simulink model "mars_rover_ex_1b_22b"  (R2022b)
settings: Solver=ode23t  StartTime=0.0  StopTime=Rover.simStopTimeEx1b  FixedStep=1e-2  MaxStep=0.05  RelTol=1e-3  AbsTol=1e-3  EnableMultiTasking=on
StartFcn:
  | mars_rover_ex1b_sim_callback
model workspace (MATLAB code in the model file):
  | addpath("mars_rover_helpers");
  | % Load Rover Arm model for IK
  | mdlpath = ['mars_rover_data',filesep,'mars_rover_arm'];
  | load_system(mdlpath);
  | 
  | imdata = zeros(3,3,3);
  | 
  | % Temp
  | Kp_steer = 1;
  | Ki_steer = 1;
  | Kd_steer = 1;
  | 
  | Kp = 1;
  | Ki = 1;
  | Kd = 1;
values from neighbouring files (symbols this model uses):
  cam_base_angle = 0    [mars_rover_params.m]
  cam_target_angle = 20    [mars_rover_params.m]
  mapData = false(197,200)    [mars_rover_params.m]    (also in mars_rover_startup.m)
  roverPath = app.rover_path    [NavigateOnMars.m]    (also in mars_rover_params.m = rover_path1)
undefined symbols (not defined in the file or in its folder): Arm, armJointAng, armJointTrqs, cameraData, eeConfig, pose, Rover, sampleLocation, steerAng, steerTrqs, Terrain, vSpeed, Wheel1_G, Wheel2_G, Wheel3_G, Wheel4_G, Wheel5_G, Wheel6_G, wheelTrqs, wSpeeds, X, Y, Z
libraries: sm_lib x238, nesl_utility x80, slpidlib x3, simulink x3, simulink_extras x2, robotcorelib x1, robotalgslib x1
(part 5 of 9)

== system mars_rover_ex_1b_22b/Perception/navCamSubsystem/rsm_lower_mast_2_RIGID ==
  note: 15 deg offset
  Cylindrical Solid : sm_lib/Body Elements/Cylindrical Solid  GraphicAmbientColor=[0.15 0.15 0.15 1.0]  BasedOnType=Density  CenterOfMass=[0 0 0]  CenterOfMassUnits=m  GraphicDiffuseColor=[1 1 0.8]  CylinderLength=3.5/10  CylinderLengthUnits=m  CylinderRadius=0.4/10  CylinderRadiusUnits=m  Density=1000  DensityUnits=kg/m^3  DoExposeReferenceFrame=on  GraphicEmissiveColor=[0.0 0.0 0.0 1.0]  ExportEntireGeometry=off  SerializedFrames=<Frames><Frame><Id>Frame1</Id><Value><Name>F1</Name><Origin><Source>GeometricFeature</Source><FeatureName>bottom surface</FeatureName></Origin><PrimaryAxis><DefinedDirection>+Z</DefinedDirection><Source>ReferenceFrame</Source><SourceDirection>+X</SourceDirection><FeatureName></FeatureName></PrimaryAxis><SecondaryAxis><DefinedDirection>+X</DefinedDirection><Source>ReferenceFrame</Source><SourceDirection>+Z</SourceDirection><FeatureName></FeatureName></SecondaryAxis></Value></Frame><Frame><Id>Frame2</Id><Value><Name>F2</Name><Origin><Source>GeometricFeature</Source><FeatureName>top surface</FeatureName></Origin><PrimaryAxis><DefinedDirection>+Z</DefinedDirection><Source>ReferenceFrame</Source><SourceDirection>+Z</SourceDirection><FeatureName></FeatureName></PrimaryAxis><SecondaryAxis><DefinedDirection>+X</DefinedDirection><Source>ReferenceFrame</Source><SourceDirection>+X</SourceDirection><FeatureName></FeatureName></SecondaryAxis></Value></Frame></Frames>  MarkerShape=Sphere  MarkerSize=10  GraphicType=FromGeometry  InertiaType=CalculateFromGeometry  Mass=1  MassUnits=kg  MomentsOfInertia=[1 1 1]  MomentsOfInertiaUnits=kg*m^2  GraphicOpacity=1.0  ProductsOfInertia=[0 0 0]  ProductsOfInertiaUnits=kg*m^2  GraphicShininess=75  GraphicSpecularColor=[0.5 0.5 0.5 1.0]  GraphicVisPropType=SimpleVisualProperties
  Cylindrical Solid1 : sm_lib/Body Elements/Cylindrical Solid  GraphicAmbientColor=[0.15 0.15 0.15 1.0]  BasedOnType=Density  CenterOfMass=[0 0 0]  CenterOfMassUnits=m  GraphicDiffuseColor=[1 1 0.8]  CylinderLength=0.85/10  CylinderLengthUnits=m  CylinderRadius=0.6/10  CylinderRadiusUnits=m  Density=1000  DensityUnits=kg/m^3  DoExposeReferenceFrame=on  GraphicEmissiveColor=[0.0 0.0 0.0 1.0]  ExportEntireGeometry=off  SerializedFrames=<Frames><Frame><Id>Frame1</Id><Value><Name>F1</Name><Origin><Source>GeometricFeature</Source><FeatureName>bottom surface</FeatureName></Origin><PrimaryAxis><DefinedDirection>+Z</DefinedDirection><Source>ReferenceFrame</Source><SourceDirection>+Z</SourceDirection><FeatureName></FeatureName></PrimaryAxis><SecondaryAxis><DefinedDirection>+X</DefinedDirection><Source>ReferenceFrame</Source><SourceDirection>+X</SourceDirection><FeatureName></FeatureName></SecondaryAxis></Value></Frame></Frames>  MarkerShape=Sphere  MarkerSize=10  GraphicType=FromGeometry  InertiaType=CalculateFromGeometry  Mass=1  MassUnits=kg  MomentsOfInertia=[1 1 1]  MomentsOfInertiaUnits=kg*m^2  GraphicOpacity=1.0  ProductsOfInertia=[0 0 0]  ProductsOfInertiaUnits=kg*m^2  GraphicShininess=75  GraphicSpecularColor=[0.5 0.5 0.5 1.0]  GraphicVisPropType=SimpleVisualProperties
  Cylindrical Solid2 : sm_lib/Body Elements/Cylindrical Solid  GraphicAmbientColor=[0.15 0.15 0.15 1.0]  BasedOnType=Density  CenterOfMass=[0 0 0]  CenterOfMassUnits=m  GraphicDiffuseColor=[1 1 0.8]  CylinderLength=0.2/10  CylinderLengthUnits=m  CylinderRadius=0.7/10  CylinderRadiusUnits=m  Density=1000  DensityUnits=kg/m^3  DoExposeReferenceFrame=on  GraphicEmissiveColor=[0.0 0.0 0.0 1.0]  ExportEntireGeometry=off  SerializedFrames=<Frames><Frame><Id>Frame1</Id><Value><Name>F1</Name><Origin><Source>GeometricFeature</Source><FeatureName>top surface</FeatureName></Origin><PrimaryAxis><DefinedDirection>+Z</DefinedDirection><Source>ReferenceFrame</Source><SourceDirection>+Z</SourceDirection><FeatureName></FeatureName></PrimaryAxis><SecondaryAxis><DefinedDirection>+X</DefinedDirection><Source>ReferenceFrame</Source><SourceDirection>+X</SourceDirection><FeatureName></FeatureName></SecondaryAxis></Value></Frame></Frames>  MarkerShape=Sphere  MarkerSize=10  GraphicType=FromGeometry  InertiaType=CalculateFromGeometry  Mass=1  MassUnits=kg  MomentsOfInertia=[1 1 1]  MomentsOfInertiaUnits=kg*m^2  GraphicOpacity=1.0  ProductsOfInertia=[0 0 0]  ProductsOfInertiaUnits=kg*m^2  GraphicShininess=75  GraphicSpecularColor=[0.5 0.5 0.5 1.0]  GraphicVisPropType=SimpleVisualProperties
  Cylindrical Solid3 : sm_lib/Body Elements/Cylindrical Solid  GraphicAmbientColor=[0.15 0.15 0.15 1.0]  BasedOnType=Density  CenterOfMass=[0 0 0]  CenterOfMassUnits=m  GraphicDiffuseColor=[1 1 0.8]  CylinderLength=1.25/10  CylinderLengthUnits=m  CylinderRadius=0.15/10  CylinderRadiusUnits=m  Density=2000  DensityUnits=kg/m^3  DoExposeReferenceFrame=off  GraphicEmissiveColor=[0.0 0.0 0.0 1.0]  ExportEntireGeometry=off  SerializedFrames=<Frames><Frame><Id>Frame1</Id><Value><Name>F1</Name><Origin><Source>GeometricFeature</Source><FeatureName>bottom surface</FeatureName></Origin><PrimaryAxis><DefinedDirection>+Z</DefinedDirection><Source>ReferenceFrame</Source><SourceDirection>+Z</SourceDirection><FeatureName></FeatureName></PrimaryAxis><SecondaryAxis><DefinedDirection>+X</DefinedDirection><Source>ReferenceFrame</Source><SourceDirection>+X</SourceDirection><FeatureName></FeatureName></SecondaryAxis></Value></Frame></Frames>  MarkerShape=Sphere  MarkerSize=10  GraphicType=FromGeometry  InertiaType=CalculateFromGeometry  Mass=1  MassUnits=kg  MomentsOfInertia=[1 1 1]  MomentsOfInertiaUnits=kg*m^2  GraphicOpacity=1.0  ProductsOfInertia=[0 0 0]  ProductsOfInertiaUnits=kg*m^2  GraphicShininess=75  GraphicSpecularColor=[0.5 0.5 0.5 1.0]  GraphicVisPropType=SimpleVisualProperties
  Cylindrical Solid4 : sm_lib/Body Elements/Cylindrical Solid  GraphicAmbientColor=[0.15 0.15 0.15 1.0]  BasedOnType=Density  CenterOfMass=[0 0 0]  CenterOfMassUnits=m  GraphicDiffuseColor=[1 1 0.8]  CylinderLength=1.5/10  CylinderLengthUnits=m  CylinderRadius=0.15/10  CylinderRadiusUnits=m  Density=2000  DensityUnits=kg/m^3  DoExposeReferenceFrame=off  GraphicEmissiveColor=[0.0 0.0 0.0 1.0]  ExportEntireGeometry=off  SerializedFrames=<Frames><Frame><Id>Frame1</Id><Value><Name>F1</Name><Origin><Source>GeometricFeature</Source><FeatureName>bottom surface</FeatureName></Origin><PrimaryAxis><DefinedDirection>+Z</DefinedDirection><Source>ReferenceFrame</Source><SourceDirection>+Z</SourceDirection><FeatureName></FeatureName></PrimaryAxis><SecondaryAxis><DefinedDirection>+X</DefinedDirection><Source>ReferenceFrame</Source><SourceDirection>+X</SourceDirection><FeatureName></FeatureName></SecondaryAxis></Value></Frame></Frames>  MarkerShape=Sphere  MarkerSize=10  GraphicType=FromGeometry  InertiaType=CalculateFromGeometry  Mass=1  MassUnits=kg  MomentsOfInertia=[1 1 1]  MomentsOfInertiaUnits=kg*m^2  GraphicOpacity=1.0  ProductsOfInertia=[0 0 0]  ProductsOfInertiaUnits=kg*m^2  GraphicShininess=75  GraphicSpecularColor=[0.5 0.5 0.5 1.0]  GraphicVisPropType=SimpleVisualProperties
  Rigid Transform : sm_lib/Frames and Transforms/Rigid Transform  TranslationMethod=StandardAxis  TranslationStandardOffset=-0.55  TranslationLengthUnit=cm  TranslationStandardAxis=+X  TranslationCartesianOffset=[0 0 0]  TranslationROffset=0  TranslationROffsetUnits=m  TranslationZOffset=0  TranslationZOffsetUnits=m  TranslationThetaOffset=0  TranslationThetaOffsetUnits=deg  RotationMethod=None  RotationAngleUnits=deg  RotationStandardAxis=+X  RotationAngle=75  RotationArbitraryAxis=[0 0 1]  FollAlignAxisA=+X  BaseAlignAxisA=+Y  FollAlignAxisB=+Y  BaseAlignAxisB=+Z  RotationSequenceAxes=FollowerAxes  RotationSequence=XYX  RotationSequenceAngles=[0 0 0]  RotationSequenceAnglesUnits=deg  RotationMatrix=[1 0 0; 0 1 0; 0 0 1]  Quaternion=[1 0 0 0]
  Rigid Transform1 : sm_lib/Frames and Transforms/Rigid Transform  TranslationMethod=Cartesian  TranslationStandardOffset=-0.55  TranslationLengthUnit=cm  TranslationStandardAxis=+X  TranslationCartesianOffset=[0 -0.3 1]  TranslationROffset=0  TranslationROffsetUnits=m  TranslationZOffset=0  TranslationZOffsetUnits=m  TranslationThetaOffset=0  TranslationThetaOffsetUnits=deg  RotationMethod=StandardAxis  RotationAngleUnits=deg  RotationStandardAxis=+X  RotationAngle=45  RotationArbitraryAxis=[0 0 1]  FollAlignAxisA=+X  BaseAlignAxisA=+Y  FollAlignAxisB=+Y  BaseAlignAxisB=+Z  RotationSequenceAxes=FollowerAxes  RotationSequence=ZYZ  RotationSequenceAngles=[0 -90 0]  RotationSequenceAnglesUnits=deg  RotationMatrix=[1 0 0; 0 1 0; 0 0 1]  Quaternion=[1 0 0 0]
  Rigid Transform2 : sm_lib/Frames and Transforms/Rigid Transform  TranslationMethod=Cartesian  TranslationStandardOffset=-0.55  TranslationLengthUnit=cm  TranslationStandardAxis=+X  TranslationCartesianOffset=[0 0.3 1]  TranslationROffset=0  TranslationROffsetUnits=m  TranslationZOffset=0  TranslationZOffsetUnits=m  TranslationThetaOffset=0  TranslationThetaOffsetUnits=deg  RotationMethod=StandardAxis  RotationAngleUnits=deg  RotationStandardAxis=+X  RotationAngle=-45  RotationArbitraryAxis=[0 0 1]  FollAlignAxisA=+X  BaseAlignAxisA=+Y  FollAlignAxisB=+Y  BaseAlignAxisB=+Z  RotationSequenceAxes=FollowerAxes  RotationSequence=ZYZ  RotationSequenceAngles=[0 90 0]  RotationSequenceAnglesUnits=deg  RotationMatrix=[1 0 0; 0 1 0; 0 0 1]  Quaternion=[1 0 0 0]
  Bottom : PMIOPort  Side=Left
  Top : PMIOPort  Port=2  Side=Right
  connections:
  Cylindrical Solid2/RConn1 -- Cylindrical Solid/LConn2
  Bottom/RConn1 -- Cylindrical Solid1/LConn1
  Top/RConn1 -- Cylindrical Solid2/LConn1
  Cylindrical Solid4/LConn1 -- Rigid Transform1/RConn1
  Rigid Transform/RConn1 -- Cylindrical Solid1/RConn1
  Rigid Transform/LConn1 -- Cylindrical Solid/LConn1
  Cylindrical Solid/RConn1 -- Rigid Transform2/LConn1 -- Rigid Transform1/LConn1
  Cylindrical Solid3/LConn1 -- Rigid Transform2/RConn1

== system mars_rover_ex_1b_22b/Perception/navCamSubsystem/rsm_outer_ring_1_RIGID ==
  Cylindrical Solid1 : sm_lib/Body Elements/Cylindrical Solid  GraphicAmbientColor=[0.15 0.15 0.15 1.0]  BasedOnType=Density  CenterOfMass=[0 0 0]  CenterOfMassUnits=m  GraphicDiffuseColor=[0.2 0.2 0.2]  CylinderLength=0.5/10  CylinderLengthUnits=m  CylinderRadius=0.9/10  CylinderRadiusUnits=m  Density=2000  DensityUnits=kg/m^3  DoExposeReferenceFrame=off  GraphicEmissiveColor=[0.0 0.0 0.0 1.0]  ExportEntireGeometry=off  SerializedFrames=<Frames><Frame><Id>Frame1</Id><Value><Name>F1</Name><Origin><Source>GeometricFeature</Source><FeatureName>bottom surface</FeatureName></Origin><PrimaryAxis><DefinedDirection>+Z</DefinedDirection><Source>ReferenceFrame</Source><SourceDirection>+Z</SourceDirection><FeatureName></FeatureName></PrimaryAxis><SecondaryAxis><DefinedDirection>+X</DefinedDirection><Source>ReferenceFrame</Source><SourceDirection>+X</SourceDirection><FeatureName></FeatureName></SecondaryAxis></Value></Frame><Frame><Id>Frame2</Id><Value><Name>F2</Name><Origin><Source>GeometricFeature</Source><FeatureName>top surface</FeatureName></Origin><PrimaryAxis><DefinedDirection>+Z</DefinedDirection><Source>ReferenceFrame</Source><SourceDirection>+Z</SourceDirection><FeatureName></FeatureName></PrimaryAxis><SecondaryAxis><DefinedDirection>+X</DefinedDirection><Source>ReferenceFrame</Source><SourceDirection>+X</SourceDirection><FeatureName></FeatureName></SecondaryAxis></Value></Frame></Frames>  MarkerShape=Sphere  MarkerSize=10  GraphicType=FromGeometry  InertiaType=CalculateFromGeometry  Mass=1  MassUnits=kg  MomentsOfInertia=[1 1 1]  MomentsOfInertiaUnits=kg*m^2  GraphicOpacity=1.0  ProductsOfInertia=[0 0 0]  ProductsOfInertiaUnits=kg*m^2  GraphicShininess=75  GraphicSpecularColor=[0.5 0.5 0.5 1.0]  GraphicVisPropType=SimpleVisualProperties
  F1 : PMIOPort  Side=Left
  F : PMIOPort  Port=2  Side=Left
  connections:
  F1/RConn1 -- Cylindrical Solid1/RConn1
  F/RConn1 -- Cylindrical Solid1/LConn1

== system mars_rover_ex_1b_22b/Perception/navCamSubsystem/rsm_upper_mast_1_RIGID ==
  In1 : Inport
  CamUpDown : sm_lib/Joints/Revolute Joint  JointMode=Normal  SenseConstraintForce=off  SenseConstraintForceX=off  SenseConstraintForceY=off  SenseConstraintForceZ=off  SenseConstraintTorque=off  SenseConstraintTorqueX=off  SenseConstraintTorqueY=off  SenseConstraintTorqueZ=off  SenseTotalForce=off  SenseTotalForceX=off  SenseTotalForceY=off  SenseTotalForceZ=off  SenseTotalTorque=off  SenseTotalTorqueX=off  SenseTotalTorqueY=off  SenseTotalTorqueZ=off  CompositeWrenchDir=FollowerOnBase  CompositeWrenchFrame=BaseFrame  EquilibriumPosition=0  EquilibriumPositionUnits=deg  SpringStiffness=0  SpringStiffnessUnits=N*m/deg  DampingCoefficient=0  DampingCoefficientUnits=N*m/(deg/s)  TorqueActuationMode=ComputedTorque  MotionActuationMode=InputMotion  SensePosition=off  SenseVelocity=off  SenseAcceleration=off  SenseTorqueForce=off  SenseLowerLimitTorqueForce=off  SenseUpperLimitTorqueForce=off  LowerLimitSpecify=off  LowerLimitBound=-90  LowerLimitBoundUnits=deg  LowerLimitStiffness=1e4  LowerLimitStiffnessUnits=N*m/deg  LowerLimitDamping=10  LowerLimitDampingUnits=N*m/(deg/s)  LowerLimitTransitionRegionWidth=0.1  LowerLimitTransitionRegionWidthUnits=deg  UpperLimitSpecify=off  UpperLimitBound=90  UpperLimitBoundUnits=deg  UpperLimitStiffness=1e4  UpperLimitStiffnessUnits=N*m/deg  UpperLimitDamping=10  UpperLimitDampingUnits=N*m/(deg/s)  UpperLimitTransitionRegionWidth=0.1  UpperLimitTransitionRegionWidthUnits=deg  PositionTargetSpecify=on  PositionTargetPriority=High  PositionTargetValue=30  PositionTargetValueUnits=deg  VelocityTargetSpecify=off  VelocityTargetPriority=High  VelocityTargetValue=0  VelocityTargetValueUnits=deg/s
  Cylindrical Solid : sm_lib/Body Elements/Cylindrical Solid  GraphicAmbientColor=[0.15 0.15 0.15 1.0]  BasedOnType=Density  CenterOfMass=[0 0 0]  CenterOfMassUnits=m  GraphicDiffuseColor=[1 1 0.8]  CylinderLength=1.8/10  CylinderLengthUnits=m  CylinderRadius=0.4/10  CylinderRadiusUnits=m  Density=2000  DensityUnits=kg/m^3  DoExposeReferenceFrame=off  GraphicEmissiveColor=[0.0 0.0 0.0 1.0]  ExportEntireGeometry=off  SerializedFrames=<Frames><Frame><Id>Frame1</Id><Value><Name>F1</Name><Origin><Source>GeometricFeature</Source><FeatureName>bottom surface</FeatureName></Origin><PrimaryAxis><DefinedDirection>+Z</DefinedDirection><Source>ReferenceFrame</Source><SourceDirection>+X</SourceDirection><FeatureName></FeatureName></PrimaryAxis><SecondaryAxis><DefinedDirection>+X</DefinedDirection><Source>ReferenceFrame</Source><SourceDirection>+Z</SourceDirection><FeatureName></FeatureName></SecondaryAxis></Value></Frame><Frame><Id>Frame2</Id><Value><Name>F2</Name><Origin><Source>GeometricFeature</Source><FeatureName>top surface</FeatureName></Origin><PrimaryAxis><DefinedDirection>+Z</DefinedDirection><Source>ReferenceFrame</Source><SourceDirection>-Z</SourceDirection><FeatureName></FeatureName></PrimaryAxis><SecondaryAxis><DefinedDirection>+X</DefinedDirection><Source>ReferenceFrame</Source><SourceDirection>+X</SourceDirection><FeatureName></FeatureName></SecondaryAxis></Value></Frame></Frames>  MarkerShape=Sphere  MarkerSize=10  GraphicType=FromGeometry  InertiaType=CalculateFromGeometry  Mass=1  MassUnits=kg  MomentsOfInertia=[1 1 1]  MomentsOfInertiaUnits=kg*m^2  GraphicOpacity=1.0  ProductsOfInertia=[0 0 0]  ProductsOfInertiaUnits=kg*m^2  GraphicShininess=75  GraphicSpecularColor=[0.5 0.5 0.5 1.0]  GraphicVisPropType=SimpleVisualProperties
  Cylindrical Solid1 : sm_lib/Body Elements/Cylindrical Solid  GraphicAmbientColor=[0.15 0.15 0.15 1.0]  BasedOnType=Density  CenterOfMass=[0 0 0]  CenterOfMassUnits=m  GraphicDiffuseColor=[1 1 0.8]  CylinderLength=0.85/10  CylinderLengthUnits=m  CylinderRadius=0.6/10  CylinderRadiusUnits=m  Density=2000  DensityUnits=kg/m^3  DoExposeReferenceFrame=on  GraphicEmissiveColor=[0.0 0.0 0.0 1.0]  ExportEntireGeometry=off  SerializedFrames=<Frames><Frame><Id>Frame1</Id><Value><Name>F1</Name><Origin><Source>GeometricFeature</Source><FeatureName>bottom surface</FeatureName></Origin><PrimaryAxis><DefinedDirection>+Z</DefinedDirection><Source>ReferenceFrame</Source><SourceDirection>+Z</SourceDirection><FeatureName></FeatureName></PrimaryAxis><SecondaryAxis><DefinedDirection>+X</DefinedDirection><Source>ReferenceFrame</Source><SourceDirection>+X</SourceDirection><FeatureName></FeatureName></SecondaryAxis></Value></Frame></Frames>  MarkerShape=Sphere  MarkerSize=10  GraphicType=FromGeometry  InertiaType=CalculateFromGeometry  Mass=1  MassUnits=kg  MomentsOfInertia=[1 1 1]  MomentsOfInertiaUnits=kg*m^2  GraphicOpacity=1.0  ProductsOfInertia=[0 0 0]  ProductsOfInertiaUnits=kg*m^2  GraphicShininess=75  GraphicSpecularColor=[0.5 0.5 0.5 1.0]  GraphicVisPropType=SimpleVisualProperties
  Rigid Transform : sm_lib/Frames and Transforms/Rigid Transform  TranslationMethod=StandardAxis  TranslationStandardOffset=-0.55  TranslationLengthUnit=cm  TranslationStandardAxis=+X  TranslationCartesianOffset=[0 0 0]  TranslationROffset=0  TranslationROffsetUnits=m  TranslationZOffset=0  TranslationZOffsetUnits=m  TranslationThetaOffset=0  TranslationThetaOffsetUnits=deg  RotationMethod=None  RotationAngleUnits=deg  RotationStandardAxis=+X  RotationAngle=180+120  RotationArbitraryAxis=[0 0 1]  FollAlignAxisA=+X  BaseAlignAxisA=+Y  FollAlignAxisB=+Y  BaseAlignAxisB=+Z  RotationSequenceAxes=FollowerAxes  RotationSequence=XYX  RotationSequenceAngles=[0 0 0]  RotationSequenceAnglesUnits=deg  RotationMatrix=[1 0 0; 0 1 0; 0 0 1]  Quaternion=[1 0 0 0]
  Simulink-PS Converter : nesl_utility/Simulink-PS Converter  PhysicalDomain=network_engine_domain  SubClassName=ps_input  LeftPortType=input  RightPortType=output  PseudoPeriodic=off  Frequencies=[]  NoiseDistribution=none  NoiseParameters=[]  Unit=deg  AffineConversion=off  FilteringAndDerivatives=filter  SimscapeFilterOrder=2  InputFilterTimeConstant=0.001  UdotUserProvided=0
  F : PMIOPort  Side=Left
  F1 : PMIOPort  Port=2  Side=Right
  wires:
  In1/1 -> Simulink-PS Converter/1
  connections:
  Cylindrical Solid1/LConn1 -- F1/RConn1
  F/RConn1 -- Cylindrical Solid/RConn1
  CamUpDown/RConn1 -- Cylindrical Solid1/RConn1
  Rigid Transform/LConn1 -- Cylindrical Solid/LConn1
  Rigid Transform/RConn1 -- CamUpDown/LConn1
  Simulink-PS Converter/RConn1 -- CamUpDown/LConn2

== system mars_rover_ex_1b_22b/Perception/sceneViewer/Left ==
  Constant6 : Constant  Value=cam_target_angle
  LCam : MATLAB Function  TreatAsAtomicUnit=on
  PS-Simulink Converter{,1..3} (4 alike) : nesl_utility/PS-Simulink Converter  PhysicalDomain=network_engine_domain  SubClassName=ps_output  LeftPortType=input  RightPortType=output  PseudoPeriodic=off  Frequencies=[]  VectorFormat=inherit  Unit=inherit  AffineConversion=off
  Terminator{,1..3} (4 alike) : Terminator
  Transform Sensor : sm_lib/Frames and Transforms/Transform Sensor  MeasurementFrame=World  SenseAngle=off  SenseAxis=off  SenseQ=off  SenseR=on  SenseRotationSequence=off  RotationSequence=XYX  SenseOmegaX=off  SenseOmegaY=off  SenseOmegaZ=off  SenseQDot=off  SenseRDot=off  SenseAlphaX=off  SenseAlphaY=off  SenseAlphaZ=off  SenseQDDot=off  SenseRDDot=off  SenseX=on  SenseY=on  SenseZ=on  SenseRad=off  SenseAzim=off  SenseDist=off  SenseInc=off  SenseXDot=off  SenseYDot=off  SenseZDot=off  SenseRadDot=off  SenseAzimDot=off  SenseDistDot=off  SenseIncDot=off  SenseXDDot=off  SenseYDDot=off  SenseZDDot=off  SenseRadDDot=off  SenseAzimDDot=off  SenseDistDDot=off  SenseIncDDot=off
  World Frame : sm_lib/Frames and Transforms/World Frame
  camFrame : PMIOPort  Side=Right
  wires:
  LCam/4(Camera_target_ang) -> Terminator3/1
  LCam/3(Camera_rot) -> Terminator2/1
  PS-Simulink Converter2/1 -> LCam/4(z)
  Constant6/1 -> LCam/5(target_ang)
  PS-Simulink Converter3/1 -> LCam/1(rot_mat)
  PS-Simulink Converter/1 -> LCam/2(x)
  PS-Simulink Converter1/1 -> LCam/3(y)
  LCam/1(Camera_Z_ang) -> Terminator/1
  LCam/2(Camera_pos) -> Terminator1/1
  connections:
  camFrame/RConn1 -- Transform Sensor/RConn1
  Transform Sensor/RConn5 -- PS-Simulink Converter2/LConn1
  World Frame/RConn1 -- Transform Sensor/LConn1
  Transform Sensor/RConn2 -- PS-Simulink Converter3/LConn1
  Transform Sensor/RConn3 -- PS-Simulink Converter/LConn1
  Transform Sensor/RConn4 -- PS-Simulink Converter1/LConn1

== system mars_rover_ex_1b_22b/Perception/sceneViewer/Right ==
  Constant6 : Constant  Value=cam_target_angle
  PS-Simulink Converter{,1..3} (4 alike) : nesl_utility/PS-Simulink Converter  PhysicalDomain=network_engine_domain  SubClassName=ps_output  LeftPortType=input  RightPortType=output  PseudoPeriodic=off  Frequencies=[]  VectorFormat=inherit  Unit=inherit  AffineConversion=off
  RCam : MATLAB Function  TreatAsAtomicUnit=on
  Terminator{,1..3} (4 alike) : Terminator
  Transform Sensor : sm_lib/Frames and Transforms/Transform Sensor  MeasurementFrame=World  SenseAngle=off  SenseAxis=off  SenseQ=off  SenseR=on  SenseRotationSequence=off  RotationSequence=XYX  SenseOmegaX=off  SenseOmegaY=off  SenseOmegaZ=off  SenseQDot=off  SenseRDot=off  SenseAlphaX=off  SenseAlphaY=off  SenseAlphaZ=off  SenseQDDot=off  SenseRDDot=off  SenseX=on  SenseY=on  SenseZ=on  SenseRad=off  SenseAzim=off  SenseDist=off  SenseInc=off  SenseXDot=off  SenseYDot=off  SenseZDot=off  SenseRadDot=off  SenseAzimDot=off  SenseDistDot=off  SenseIncDot=off  SenseXDDot=off  SenseYDDot=off  SenseZDDot=off  SenseRadDDot=off  SenseAzimDDot=off  SenseDistDDot=off  SenseIncDDot=off
  World Frame : sm_lib/Frames and Transforms/World Frame
  camFrame : PMIOPort  Side=Right
  wires:
  RCam/4(Camera_target_ang) -> Terminator3/1
  RCam/3(Camera_rot) -> Terminator2/1
  RCam/1(Camera_Z_ang) -> Terminator/1
  PS-Simulink Converter2/1 -> RCam/4(z)
  PS-Simulink Converter3/1 -> RCam/1(rot_mat)
  PS-Simulink Converter/1 -> RCam/2(x)
  Constant6/1 -> RCam/5(target_ang)
  PS-Simulink Converter1/1 -> RCam/3(y)
  RCam/2(Camera_pos) -> Terminator1/1
  connections:
  camFrame/RConn1 -- Transform Sensor/RConn1
  Transform Sensor/RConn2 -- PS-Simulink Converter3/LConn1
  Transform Sensor/RConn3 -- PS-Simulink Converter/LConn1
  Transform Sensor/RConn4 -- PS-Simulink Converter1/LConn1
  World Frame/RConn1 -- Transform Sensor/LConn1
  Transform Sensor/RConn5 -- PS-Simulink Converter2/LConn1

== system mars_rover_ex_1b_22b/Perception/sceneViewer/Stereo_Left ==
  Input : Inport
  Constant : Constant  Value=Terrain.xg
  Constant1 : Constant  Value=Terrain.yg
  Constant2 : Constant  Value=Terrain.z_heights
  Constant3 : Constant  Value=roverPath.x
  Constant4 : Constant  Value=roverPath.y
  Constant5 : Constant  Value=roverPath.z
  Constant6 : Constant  Value=cam_target_angle
  Constant7 : Constant  Value=Terrain.znew
  Mux : Mux  Inputs=3
  PS-Simulink Converter{,1..3} (4 alike) : nesl_utility/PS-Simulink Converter  PhysicalDomain=network_engine_domain  SubClassName=ps_output  LeftPortType=input  RightPortType=output  PseudoPeriodic=off  Frequencies=[]  VectorFormat=inherit  Unit=inherit  AffineConversion=off
  Transform Sensor : sm_lib/Frames and Transforms/Transform Sensor  MeasurementFrame=World  SenseAngle=off  SenseAxis=off  SenseQ=off  SenseR=on  SenseRotationSequence=off  RotationSequence=XYX  SenseOmegaX=off  SenseOmegaY=off  SenseOmegaZ=off  SenseQDot=off  SenseRDot=off  SenseAlphaX=off  SenseAlphaY=off  SenseAlphaZ=off  SenseQDDot=off  SenseRDDot=off  SenseX=on  SenseY=on  SenseZ=on  SenseRad=off  SenseAzim=off  SenseDist=off  SenseInc=off  SenseXDot=off  SenseYDot=off  SenseZDot=off  SenseRadDot=off  SenseAzimDot=off  SenseDistDot=off  SenseIncDot=off  SenseXDDot=off  SenseYDDot=off  SenseZDDot=off  SenseRadDDot=off  SenseAzimDDot=off  SenseDistDDot=off  SenseIncDDot=off
  World Frame : sm_lib/Frames and Transforms/World Frame
  drawScene : Subsystem
  theta_act : MATLAB Function  TreatAsAtomicUnit=on
  B : PMIOPort  Side=Left
  im_left : Outport
  wires:
  PS-Simulink Converter2/1 -> Mux/3
  Mux/1 -> drawScene/2(Camera_pos)
  PS-Simulink Converter/1 -> Mux/1
  PS-Simulink Converter3/1 -> drawScene/3(Camera_rot), theta_act/1(u)
  PS-Simulink Converter1/1 -> Mux/2
  theta_act/1(z) -> drawScene/1(Camera_Z_ang)
  Constant6/1 -> drawScene/4(Camera_target_ang)
  Constant/1 -> drawScene/5(xg)
  Constant1/1 -> drawScene/6(yg)
  Constant2/1 -> drawScene/7(z_heights)
  Constant7/1 -> drawScene/8(znew)
  Constant3/1 -> drawScene/9(rover_path_x)
  Constant4/1 -> drawScene/10(rover_path_y)
  Constant5/1 -> drawScene/11(rover_path_z)
  drawScene/1(im) -> im_left/1
  Input/1 -> drawScene/Trigger
  connections:
  PS-Simulink Converter3/LConn1 -- Transform Sensor/RConn2
  PS-Simulink Converter2/LConn1 -- Transform Sensor/RConn5
  Transform Sensor/LConn1 -- World Frame/RConn1
  PS-Simulink Converter/LConn1 -- Transform Sensor/RConn3
  PS-Simulink Converter1/LConn1 -- Transform Sensor/RConn4
  B/RConn1 -- Transform Sensor/RConn1

== system mars_rover_ex_1b_22b/Perception/sceneViewer/Stereo_Right ==
  Input : Inport
  Constant : Constant  Value=Terrain.xg
  Constant1 : Constant  Value=Terrain.yg
  Constant2 : Constant  Value=Terrain.z_heights
  Constant3 : Constant  Value=roverPath.x
  Constant4 : Constant  Value=roverPath.y
  Constant5 : Constant  Value=roverPath.z
  Constant6 : Constant  Value=cam_target_angle
  Constant7 : Constant  Value=Terrain.znew
  Mux : Mux  Inputs=3
  PS-Simulink Converter{,1..3} (4 alike) : nesl_utility/PS-Simulink Converter  PhysicalDomain=network_engine_domain  SubClassName=ps_output  LeftPortType=input  RightPortType=output  PseudoPeriodic=off  Frequencies=[]  VectorFormat=inherit  Unit=inherit  AffineConversion=off
  Transform Sensor : sm_lib/Frames and Transforms/Transform Sensor  MeasurementFrame=World  SenseAngle=off  SenseAxis=off  SenseQ=off  SenseR=on  SenseRotationSequence=off  RotationSequence=XYX  SenseOmegaX=off  SenseOmegaY=off  SenseOmegaZ=off  SenseQDot=off  SenseRDot=off  SenseAlphaX=off  SenseAlphaY=off  SenseAlphaZ=off  SenseQDDot=off  SenseRDDot=off  SenseX=on  SenseY=on  SenseZ=on  SenseRad=off  SenseAzim=off  SenseDist=off  SenseInc=off  SenseXDot=off  SenseYDot=off  SenseZDot=off  SenseRadDot=off  SenseAzimDot=off  SenseDistDot=off  SenseIncDot=off  SenseXDDot=off  SenseYDDot=off  SenseZDDot=off  SenseRadDDot=off  SenseAzimDDot=off  SenseDistDDot=off  SenseIncDDot=off
  World Frame : sm_lib/Frames and Transforms/World Frame
  drawScene : Subsystem
  theta_act : MATLAB Function  TreatAsAtomicUnit=on
  B : PMIOPort  Side=Left
  im_right : Outport
  wires:
  PS-Simulink Converter1/1 -> Mux/2
  PS-Simulink Converter3/1 -> theta_act/1(u), drawScene/3(Camera_rot)
  PS-Simulink Converter/1 -> Mux/1
  Mux/1 -> drawScene/2(Camera_pos)
  PS-Simulink Converter2/1 -> Mux/3
  theta_act/1(z) -> drawScene/1(Camera_Z_ang)
  Constant6/1 -> drawScene/4(Camera_target_ang)
  Constant/1 -> drawScene/5(xg)
  Constant1/1 -> drawScene/6(yg)
  Constant2/1 -> drawScene/7(z_heights)
  Constant7/1 -> drawScene/8(znew)
  Constant3/1 -> drawScene/9(rover_path_x)
  Constant4/1 -> drawScene/10(rover_path_y)
  Constant5/1 -> drawScene/11(rover_path_z)
  drawScene/1(im) -> im_right/1
  Input/1 -> drawScene/Trigger
  connections:
  B/RConn1 -- Transform Sensor/RConn1
  PS-Simulink Converter1/LConn1 -- Transform Sensor/RConn4
  PS-Simulink Converter/LConn1 -- Transform Sensor/RConn3
  Transform Sensor/LConn1 -- World Frame/RConn1
  PS-Simulink Converter2/LConn1 -- Transform Sensor/RConn5
  PS-Simulink Converter3/LConn1 -- Transform Sensor/RConn2

== system mars_rover_ex_1b_22b/Control/Manipulator Control/ Trajectory Planner/Planner Subsystem ==
  note: End Effector Targets
  ActJointAngles : Inport
  SamplePosition : Inport  Port=2
  IsSamplePicked : Inport  Port=3
  IsSampleCollected : Inport  Port=4
  Enable : EnablePort
  Add2 : Sum  Inputs=+-
  Clock3 : Clock
  Clock4 : Clock
  Constant2 : Constant  Value=eeConfig.Targets
  Constant3 : Constant  Value=eeConfig.Ig
  Inverse Kinematics : MATLAB Function  TreatAsAtomicUnit=on
  Task Scheduler : MATLAB Function  TreatAsAtomicUnit=on
  Terminator2 : Terminator
  Terminator3 : Terminator
  Transpose : Math  Operator=transpose
  Trapezoidal Velocity Profile Trajectory : robotcorelib/Trapezoidal Velocity Profile Trajectory  WaypointSource=External  Waypoints=[ 0, -0.5, -1; 0, 0.5, 1 ]  NumParams=1  Parameter1=End Time  Parameter2=End Time  ParameterSource=Internal  PeakVelocity=1  Acceleration=[ 1; 2 ]  EndTime=8  AccelTime=[ 1; 2 ]  SimulateUsing=Code generation
  Unit Delay1 : UnitDelay  InitialCondition=zeros(7,6)  SampleTime=-1  HasFrameUpgradeWarning=on
  DesJointAngles : Outport
  SamplePickCmd : Outport  Port=2
  SampleDropCmd : Outport  Port=3
  stop : Outport  Port=4
  wires:
  Task Scheduler/4(sampleDropCmd) -> SampleDropCmd/1
  SamplePosition/1 -> Inverse Kinematics/3(samplePosition)
  Task Scheduler/3(samplePickCmd) -> SamplePickCmd/1
  ActJointAngles/1 -> Task Scheduler/1(actJointAngles)
  IsSamplePicked/1 -> Task Scheduler/3(samplePickSense)
  IsSampleCollected/1 -> Task Scheduler/4(sampleDropSense)
  Trapezoidal Velocity Profile Trajectory/1 -> DesJointAngles/1
  Constant3/1 -> Inverse Kinematics/2(eeIgs)
  Constant2/1 -> Inverse Kinematics/1(eePoseDes)
  Inverse Kinematics/1(jointSpaceWayPts) -> Task Scheduler/2(desJointAngles), Unit Delay1/1
  Unit Delay1/1 -> Inverse Kinematics/4(prevWayPts)
  Clock3/1 -> Task Scheduler/5(currentTime)
  Clock4/1 -> Add2/1
  Trapezoidal Velocity Profile Trajectory/3 -> Terminator3/1
  Trapezoidal Velocity Profile Trajectory/2 -> Terminator2/1
  Task Scheduler/2(reset_t) -> Add2/2
  Task Scheduler/1(wayPts) -> Transpose/1
  Transpose/1 -> Trapezoidal Velocity Profile Trajectory/2
  Add2/1 -> Trapezoidal Velocity Profile Trajectory/1
  Task Scheduler/5(stop) -> stop/1

== system mars_rover_ex_1b_22b/Control/Manipulator Control/ Trajectory Planner/SampleDropOffCmdLogic ==
  u : Inport
  Constant2 : Constant
  Data Type Conversion : DataTypeConversion  OutDataTypeStr=double  SaturateOnIntegerOverflow=off  RndMeth=Floor
  Delay : Delay
  DistanceError : MATLAB Function  Commented=on  TreatAsAtomicUnit=on
  Enabled Subsystem1 : Subsystem  TreatAsAtomicUnit=on
      settings: MinAlgLoopOccurrences=on
  Out1 : Outport
  wires:
  Delay/1 -> Out1/1
  Enabled Subsystem1/1(Out1) -> Delay/1
  Data Type Conversion/1 -> Enabled Subsystem1/Enable
  Constant2/1 -> Enabled Subsystem1/1(In1)
  u/1 -> Data Type Conversion/1

== system mars_rover_ex_1b_22b/Control/Manipulator Control/ Trajectory Planner/SampleLoc wrt arm base ==
  Enable : Inport
  SampleLoc : Inport  Port=2
  Constant2 : Constant
  Display : Display
  Enabled Subsystem1 : Subsystem  TreatAsAtomicUnit=on
      settings: MinAlgLoopOccurrences=on
  Switch : Switch  Criteria=u2 > Threshold  SaturateOnIntegerOverflow=off  InputSameDT=off
  Transpose1 : Math  Operator=transpose
  Unit Delay : UnitDelay  SampleTime=-1  HasFrameUpgradeWarning=on
  SamplePos : Outport
  wires:
  Constant2/1 -> Enabled Subsystem1/1(In1)
  SampleLoc/1 -> Switch/3
  Unit Delay/1 -> Switch/1, Transpose1/1, Display/1
  Switch/1 -> Unit Delay/1
  Enable/1 -> Enabled Subsystem1/Enable
  Enabled Subsystem1/1(Out1) -> Switch/2
  Transpose1/1 -> SamplePos/1

== system mars_rover_ex_1b_22b/Control/Manipulator Control/ Trajectory Planner/SamplePickUpCmdLogic ==
  u : Inport
  Constant2 : Constant
  Data Type Conversion : DataTypeConversion  OutDataTypeStr=double  SaturateOnIntegerOverflow=off  RndMeth=Floor
  Delay : Delay
  DistanceError : MATLAB Function  Commented=on  TreatAsAtomicUnit=on
  Enabled Subsystem1 : Subsystem  TreatAsAtomicUnit=on
      settings: MinAlgLoopOccurrences=on
  Out1 : Outport
  wires:
  u/1 -> Data Type Conversion/1
  Constant2/1 -> Enabled Subsystem1/1(In1)
  Enabled Subsystem1/1(Out1) -> Delay/1
  Delay/1 -> Out1/1
  Data Type Conversion/1 -> Enabled Subsystem1/Enable

== system mars_rover_ex_1b_22b/Control/Rover Control/Rover Path Planning And Control/Ackerman Steer Angle ==
  note: RB
  note: LB
  note: RF
  note: LF
  RoverAtGoal : Inport
  Delta : Inport  Port=2
  Ackerman Steering Angle Formulation : MATLAB Function  TreatAsAtomicUnit=on
  Clock1 : Clock
  Constant : Constant  Value=Rover.Chassis_L/2
  Constant3 : Constant  Value=6
  Constant4 : Constant  Value=Rover.Chassis_width
  Enabled Subsystem : Subsystem  TreatAsAtomicUnit=on
  Gain3 : Gain  Gain=-1
  Gain4 : Gain  Gain=-1
  Mux : Mux
  NOT : Logic  Operator=NOT  IconShape=distinctive  AllPortsSameDT=off  OutDataTypeStr=boolean
  Saturation{1..4} (4 alike) : Saturate  UpperLimit=60  LowerLimit=-60
  Switch2 : Switch  Criteria=u2 > Threshold  Threshold=1  SaturateOnIntegerOverflow=off  InputSameDT=off
  AckSteerAngs : Outport
  ChassisCenterROC : Outport  Port=2
  LWheelROC : Outport  Port=3
  RWheelROC : Outport  Port=4
  wires:
  Delta/1 -> Switch2/1
  Ackerman Steering Angle Formulation/2(RFsteerAng) -> Saturation3/1, Gain4/1
  Ackerman Steering Angle Formulation/5(R_R) -> RWheelROC/1
  Saturation4/1 -> Mux/4
  Saturation1/1 -> Mux/2
  Enabled Subsystem/1(delta) -> Ackerman Steering Angle Formulation/1(delta)
  Ackerman Steering Angle Formulation/1(LFsteerAng) -> Saturation2/1, Gain3/1
  Constant/1 -> Ackerman Steering Angle Formulation/2(L)
  Saturation3/1 -> Mux/3
  Mux/1 -> AckSteerAngs/1
  Clock1/1 -> Switch2/2
  Switch2/1 -> Enabled Subsystem/1(In1)
  Gain4/1 -> Saturation4/1
  Saturation2/1 -> Mux/1
  Constant4/1 -> Ackerman Steering Angle Formulation/3(d)
  Gain3/1 -> Saturation1/1
  Ackerman Steering Angle Formulation/4(L_R) -> LWheelROC/1
  Ackerman Steering Angle Formulation/3(R) -> ChassisCenterROC/1
  Constant3/1 -> Switch2/3
  RoverAtGoal/1 -> NOT/1
  NOT/1 -> Enabled Subsystem/Enable

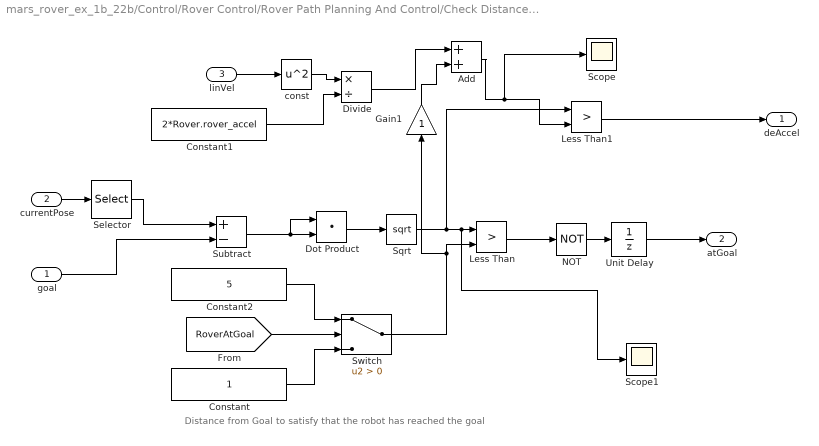
== system mars_rover_ex_1b_22b/Control/Rover Control/Rover Path Planning And Control/Check Distance To Goal ==
  note: Distance from Goal to satisfy that the robot has reached the goal
  goal : Inport
  currentPose : Inport  Port=2
  linVel : Inport  Port=3
  Add : Sum
  Constant : Constant
  Constant1 : Constant  Value=2*Rover.rover_accel
  Constant2 : Constant  Value=5
  Divide : Product  Inputs=*/
  Dot Product : DotProduct  OutDataTypeStr=Inherit: Inherit via internal rule
  Gain1 : Gain
  Less Than : RelationalOperator  Operator=>  OutDataTypeStr=boolean  RndMeth=Simplest  InputSameDT=off
  Less Than1 : RelationalOperator  Operator=>  OutDataTypeStr=boolean  RndMeth=Simplest  InputSameDT=off
  NOT : Logic  Operator=NOT  IconShape=distinctive  AllPortsSameDT=off  OutDataTypeStr=boolean
  Scope : Scope
  Scope1 : Scope
  Selector : Selector  InputPortWidth=3  IndexOptions=Index vector (dialog)  Indices=[1 2]  OutputSizes=1
  Sqrt : Sqrt
  Subtract : Sum  Inputs=+-
  Switch : Switch  Criteria=u2 > Threshold  SaturateOnIntegerOverflow=off  InputSameDT=off
  Unit Delay : UnitDelay  SampleTime=-1  HasFrameUpgradeWarning=on
  const : Math  Operator=square
  deAccel : Outport
  atGoal : Outport  Port=2
  wires:
  goal/1 -> Subtract/2
  Dot Product/1 -> Sqrt/1
  Switch/1 -> Gain1/1, Less Than/2
  Sqrt/1 -> Scope1/1, Less Than/1, Less Than1/1
  Subtract/1 -> Dot Product/1, Dot Product/2
  currentPose/1 -> Selector/1
  linVel/1 -> const/1
  const/1 -> Divide/1
  Constant1/1 -> Divide/2
  Less Than1/1 -> deAccel/1
  Add/1 -> Less Than1/2, Scope/1
  Divide/1 -> Add/1
  Gain1/1 -> Add/2
  Less Than/1 -> NOT/1
  NOT/1 -> Unit Delay/1
  Unit Delay/1 -> atGoal/1
  [RoverAtGoal] -> Switch/2
  Constant/1 -> Switch/3
  Constant2/1 -> Switch/1
  Selector/1 -> Subtract/1

== system mars_rover_ex_1b_22b/Control/Rover Control/Rover Path Planning And Control/Target Dir To Bicycle Steer Angle ==
  TargetDir : Inport
  Bicycle length : Constant  Value=L
  Constant : Constant  Value=2
  Lookahead distance : Constant  Value=ld
  Product : Product
  Product1 : Product
  Rad2Deg : MATLAB Function  TreatAsAtomicUnit=on
  Sine Wave : Sin  TimeSource=Use external signal  SampleTime=0
  Trigonometric Function : Trigonometry  Operator=atan2
  BicycleSteerAng : Outport
  wires:
  Sine Wave/1 -> Product1/2
  Bicycle length/1 -> Product/2
  Constant/1 -> Product/1
  Product/1 -> Product1/1
  Product1/1 -> Trigonometric Function/1
  Trigonometric Function/1 -> Rad2Deg/1(u)
  TargetDir/1 -> Sine Wave/1
  Lookahead distance/1 -> Trigonometric Function/2
  Rad2Deg/1(y) -> BicycleSteerAng/1

== system mars_rover_ex_1b_22b/Control/Rover Control/Rover Path Planning And Control/hold ==
  In1 : Inport
  Constant9 : Constant  Value=inf
  NOT1 : Logic  Operator=NOT  IconShape=distinctive  AllPortsSameDT=off  OutDataTypeStr=boolean
  RoverStopTime : Subsystem
  Switch3 : Switch  Criteria=u2 > Threshold  SaturateOnIntegerOverflow=off  InputSameDT=off
  Unit Delay1 : UnitDelay  SampleTime=-1  HasFrameUpgradeWarning=on
  Out1 : Outport
  wires:
  Unit Delay1/1 -> Switch3/2
  RoverStopTime/1(DeAccelTime) -> Switch3/1
  Switch3/1 -> Out1/1
  NOT1/1 -> RoverStopTime/1(Enable), Unit Delay1/1
  Constant9/1 -> Switch3/3
  In1/1 -> NOT1/1

== system mars_rover_ex_1b_22b/Control/Rover Control/Steering Controller/Subsystem ==
  In : Inport
  Add1 : Sum  Inputs=+-
  Gain : Gain  Gain=1./b
  Integrator : Integrator
  out : Outport
  wires:
  Gain/1 -> out/1, Add1/2
  Integrator/1 -> Gain/1
  In/1 -> Add1/1
  Add1/1 -> Integrator/1

== system mars_rover_ex_1b_22b/Control/Rover Control/Steering Controller/Subsystem1 ==
  In : Inport
  Add1 : Sum  Inputs=+-
  Gain : Gain  Gain=1./b
  Integrator : Integrator
  out : Outport
  wires:
  Add1/1 -> Integrator/1
  In/1 -> Add1/1
  Integrator/1 -> Gain/1
  Gain/1 -> Add1/2, out/1

== system mars_rover_ex_1b_22b/Control/Rover Control/Wheel Speed Controller/Subsystem ==
  In : Inport
  Add1 : Sum  Inputs=+-
  Gain : Gain  Gain=1./b
  Integrator : Integrator
  out : Outport
  wires:
  Gain/1 -> out/1, Add1/2
  Integrator/1 -> Gain/1
  In/1 -> Add1/1
  Add1/1 -> Integrator/1

== system mars_rover_ex_1b_22b/Control/Rover Control/Wheel Speed Controller/Subsystem1 ==
  In : Inport
  Add1 : Sum  Inputs=+-
  Gain : Gain  Gain=1./b
  Integrator : Integrator
  out : Outport
  wires:
  Add1/1 -> Integrator/1
  In/1 -> Add1/1
  Integrator/1 -> Gain/1
  Gain/1 -> Add1/2, out/1

== system mars_rover_ex_1b_22b/Mars Rover Plant/Manipulator Plant Model/Rover Arm/EndEff ==
  Cylindrical Solid : sm_lib/Body Elements/Cylindrical Solid  GraphicAmbientColor=[0.15 0.15 0.15 1.0]  BasedOnType=Mass  CenterOfMass=[0 0 0]  CenterOfMassUnits=m  GraphicDiffuseColor=[0.8 0.5058824 0.40784314]  CylinderLength=0.05  CylinderLengthUnits=m  CylinderRadius=.015  CylinderRadiusUnits=m  Density=1000  DensityUnits=kg/m^3  DoExposeReferenceFrame=on  GraphicEmissiveColor=[0.0 0.0 0.0 1.0]  ExportEntireGeometry=off  SerializedFrames=<Frames/>  MarkerShape=Sphere  MarkerSize=10  GraphicType=FromGeometry  InertiaType=CalculateFromGeometry  Mass=0.1  MassUnits=kg  MomentsOfInertia=[1 1 1]  MomentsOfInertiaUnits=kg*m^2  GraphicOpacity=0.2  ProductsOfInertia=[0 0 0]  ProductsOfInertiaUnits=kg*m^2  GraphicShininess=75  GraphicSpecularColor=[0.5 0.5 0.5 1.0]  GraphicVisPropType=SimpleVisualProperties
  EndEffector : sm_lib/Frames and Transforms/Rigid Transform  TranslationMethod=Cartesian  TranslationStandardOffset=0  TranslationLengthUnit=cm  TranslationStandardAxis=+Z  TranslationCartesianOffset=[-0.1 9.15 24]  TranslationROffset=0  TranslationROffsetUnits=m  TranslationZOffset=0  TranslationZOffsetUnits=m  TranslationThetaOffset=0  TranslationThetaOffsetUnits=deg  RotationMethod=None  RotationAngleUnits=deg  RotationStandardAxis=+Z  RotationAngle=90  RotationArbitraryAxis=[1 1 1 ]  FollAlignAxisA=+X  BaseAlignAxisA=+Y  FollAlignAxisB=+Y  BaseAlignAxisB=+Z  RotationSequenceAxes=FollowerAxes  RotationSequence=XYX  RotationSequenceAngles=[0 0 0]  RotationSequenceAnglesUnits=deg  RotationMatrix=[1 0 0; 0 1 0; 0 0 1]  Quaternion=[1 0 0 0]
  ReferenceFrame : sm_lib/Frames and Transforms/Reference Frame
  Solid : sm_lib/Body Elements/File Solid  ExtGeomFileName=arm_drill.STL  UnitType=Custom  ExtGeomFileUnits=cm  StepReaderType=HEX  ExportConvexHullGeometry=off  InertiaType=CalculateFromGeometry  Mass=0  MassUnits=kg  CenterOfMass=[0 0 0]  CenterOfMassUnits=m  MomentsOfInertia=[1 1 1]  MomentsOfInertiaUnits=kg*m^2  ProductsOfInertia=[0 0 0]  ProductsOfInertiaUnits=kg*m^2  BasedOnType=Density  Density=1000  DensityUnits=kg/m^3  DoExposeReferenceFrame=on  SerializedFrames=<Frames/>  GraphicType=FromGeometry  MarkerShape=Sphere  MarkerSize=10  GraphicVisPropType=SimpleVisualProperties  GraphicDiffuseColor=[0.8 0.5058824 0.40784314]  GraphicSpecularColor=[0.15 0.15 0.15 1]  GraphicAmbientColor=[0.15 0.15 0.15 1]  GraphicEmissiveColor=[0.2 0.2 0.2 1.0]  GraphicShininess=75  GraphicOpacity=1
  Transform : sm_lib/Frames and Transforms/Rigid Transform  TranslationMethod=None  TranslationStandardOffset=90  TranslationLengthUnit=cm  TranslationStandardAxis=+X  TranslationCartesianOffset=[-5 -5 -45]  TranslationROffset=0  TranslationROffsetUnits=m  TranslationZOffset=0  TranslationZOffsetUnits=m  TranslationThetaOffset=0  TranslationThetaOffsetUnits=deg  RotationMethod=StandardAxis  RotationAngleUnits=deg  RotationStandardAxis=+X  RotationAngle=90  RotationArbitraryAxis=[1 1 1]  FollAlignAxisA=+X  BaseAlignAxisA=+Y  FollAlignAxisB=+Y  BaseAlignAxisB=+Z  RotationSequenceAxes=FollowerAxes  RotationSequence=XYX  RotationSequenceAngles=[0 0 0]  RotationSequenceAnglesUnits=deg  RotationMatrix=[1 0 0; 0 1 0; 0 0 1]  Quaternion=[1 0 0 0]
  F : PMIOPort  Side=Left
  EndEffTip2 : PMIOPort  Port=2  Side=Right
  connections:
  Cylindrical Solid/RConn1 -- EndEffTip2/RConn1 -- EndEffector/RConn1
  Transform/RConn1 -- F/RConn1
  EndEffector/LConn1 -- Transform/LConn1 -- ReferenceFrame/RConn1 -- Solid/RConn1

== system mars_rover_ex_1b_22b/Mars Rover Plant/Manipulator Plant Model/Rover Arm/Link1 ==
  Motor1_Geom : sm_lib/Body Elements/Cylindrical Solid  GraphicAmbientColor=[0.15 0.15 0.15 1.0]  BasedOnType=Density  CenterOfMass=[0 0 0]  CenterOfMassUnits=m  GraphicDiffuseColor=[0.6 0.2 0.0]  CylinderLength=8  CylinderLengthUnits=cm  CylinderRadius=6  CylinderRadiusUnits=cm  Density=1000  DensityUnits=kg/m^3  DoExposeReferenceFrame=on  GraphicEmissiveColor=[0.0 0.0 0.0 1.0]  ExportEntireGeometry=off  SerializedFrames=<Frames/>  MarkerShape=Sphere  MarkerSize=10  GraphicType=FromGeometry  InertiaType=CalculateFromGeometry  Mass=1  MassUnits=kg  MomentsOfInertia=[1 1 1]  MomentsOfInertiaUnits=kg*m^2  GraphicOpacity=1.0  ProductsOfInertia=[0 0 0]  ProductsOfInertiaUnits=kg*m^2  GraphicShininess=75  GraphicSpecularColor=[0.5 0.5 0.5 1.0]  GraphicVisPropType=SimpleVisualProperties
  Motor2_Geom : sm_lib/Body Elements/Cylindrical Solid  GraphicAmbientColor=[0.15 0.15 0.15 1.0]  BasedOnType=Density  CenterOfMass=[0 0 0]  CenterOfMassUnits=m  GraphicDiffuseColor=[0.6 0.2 0.0]  CylinderLength=8  CylinderLengthUnits=cm  CylinderRadius=6  CylinderRadiusUnits=cm  Density=1000  DensityUnits=kg/m^3  DoExposeReferenceFrame=off  GraphicEmissiveColor=[0.0 0.0 0.0 1.0]  ExportEntireGeometry=off  SerializedFrames=<Frames><Frame><Id>Frame1</Id><Value><Name>F1</Name><Origin><Source>GeometricFeature</Source><FeatureName>top surface</FeatureName></Origin><PrimaryAxis><DefinedDirection>+Z</DefinedDirection><Source>ReferenceFrame</Source><SourceDirection>+Z</SourceDirection><FeatureName></FeatureName></PrimaryAxis><SecondaryAxis><DefinedDirection>+X</DefinedDirection><Source>ReferenceFrame</Source><SourceDirection>+X</SourceDirection><FeatureName></FeatureName></SecondaryAxis></Value></Frame></Frames>  MarkerShape=Sphere  MarkerSize=10  GraphicType=FromGeometry  InertiaType=CalculateFromGeometry  Mass=1  MassUnits=kg  MomentsOfInertia=[1 1 1]  MomentsOfInertiaUnits=kg*m^2  GraphicOpacity=1.0  ProductsOfInertia=[0 0 0]  ProductsOfInertiaUnits=kg*m^2  GraphicShininess=75  GraphicSpecularColor=[0.5 0.5 0.5 1.0]  GraphicVisPropType=SimpleVisualProperties
  ReferenceFrame : sm_lib/Frames and Transforms/Reference Frame
  Rigid Transform : sm_lib/Frames and Transforms/Rigid Transform  TranslationMethod=Cartesian  TranslationStandardOffset=0  TranslationLengthUnit=cm  TranslationStandardAxis=+Z  TranslationCartesianOffset=[ 0 -4 0]  TranslationROffset=0  TranslationROffsetUnits=m  TranslationZOffset=0  TranslationZOffsetUnits=m  TranslationThetaOffset=0  TranslationThetaOffsetUnits=deg  RotationMethod=StandardAxis  RotationAngleUnits=deg  RotationStandardAxis=+X  RotationAngle=90  RotationArbitraryAxis=[0 0 1]  FollAlignAxisA=+X  BaseAlignAxisA=+Y  FollAlignAxisB=+Y  BaseAlignAxisB=+Z  RotationSequenceAxes=FollowerAxes  RotationSequence=XYX  RotationSequenceAngles=[0 0 0]  RotationSequenceAnglesUnits=deg  RotationMatrix=[1 0 0; 0 1 0; 0 0 1]  Quaternion=[1 0 0 0]
  Solid : sm_lib/Body Elements/File Solid  ExtGeomFileName=arm_azimuth_elevation.STL  UnitType=Custom  ExtGeomFileUnits=cm  StepReaderType=HEX  ExportConvexHullGeometry=off  InertiaType=CalculateFromGeometry  Mass=0  MassUnits=kg  CenterOfMass=[0 0 0]  CenterOfMassUnits=m  MomentsOfInertia=[1 1 1]  MomentsOfInertiaUnits=kg*m^2  ProductsOfInertia=[0 0 0]  ProductsOfInertiaUnits=kg*m^2  BasedOnType=Density  Density=2700  DensityUnits=kg/m^3  DoExposeReferenceFrame=on  SerializedFrames=<Frames/>  GraphicType=FromGeometry  MarkerShape=Sphere  MarkerSize=10  GraphicVisPropType=SimpleVisualProperties  GraphicDiffuseColor=[0.2 0.2 0.2]  GraphicSpecularColor=[0.5 0.5 0.5 1.0]  GraphicAmbientColor=[0.15 0.15 0.15 1.0]  GraphicEmissiveColor=[0.0 0.0 0.0 1.0]  GraphicShininess=75  GraphicOpacity=1
  Transform : sm_lib/Frames and Transforms/Rigid Transform  TranslationMethod=Cartesian  TranslationStandardOffset=0  TranslationLengthUnit=cm  TranslationStandardAxis=+Z  TranslationCartesianOffset=Arm.Link1.translation/1000  TranslationROffset=0  TranslationROffsetUnits=m  TranslationZOffset=0  TranslationZOffsetUnits=m  TranslationThetaOffset=0  TranslationThetaOffsetUnits=deg  RotationMethod=None  RotationAngleUnits=rad  RotationStandardAxis=+Z  RotationAngle=0  RotationArbitraryAxis=[0 0 0]  FollAlignAxisA=+X  BaseAlignAxisA=+Y  FollAlignAxisB=+Y  BaseAlignAxisB=+Z  RotationSequenceAxes=FollowerAxes  RotationSequence=XYX  RotationSequenceAngles=[0 0 0]  RotationSequenceAnglesUnits=deg  RotationMatrix=[1 0 0; 0 1 0; 0 0 1]  Quaternion=[1 0 0 0]
  F1 : PMIOPort  Side=Left
  F : PMIOPort  Port=2  Side=Right
  connections:
  F1/RConn1 -- Motor1_Geom/RConn1 -- Rigid Transform/RConn1
  Transform/RConn1 -- Motor2_Geom/LConn1 -- F/RConn1
  Rigid Transform/LConn1 -- Solid/RConn1 -- ReferenceFrame/RConn1 -- Transform/LConn1
